simulink model "randomControllerSim2"  (R2015b)
settings: Solver=ode45  SolverMode=SingleTasking  StartTime=0.0  StopTime=2  RelTol=1e-3
values from neighbouring files (symbols this model uses):
  B_f = 7.4e-3    (= 0.0074)    [randomController.m]
  B_w = 17.03e-6    (= 1.703e-05)    [randomController.m]
  g = 9.82    [randomController.m]
  J_f = 5.6e-3    (= 0.0056)    [randomController.m]
  J_w = 0.601e-3    (= 0.000601)    [randomController.m]
  l_f = 0.08498    [randomController.m]
  l_w = 0.093    [randomController.m]
  m_f = 0.77-m_w    (= 0.548)    [randomController.m]
  m_w = 0.222    [randomController.m]
settings Model: Creator=USUARIO  LastModifiedBy=USUARIO
settings DataIOCC: SaveFormat=Array
settings OptimizationCC: BlockReduction=off  BooleanDataType=off
settings DebuggingCC: SaveWithParameterizedLinksMsg=none  UnderspecifiedInitializationDetection=Classic  MergeDetectMultiDrivingBlocksExec=none  SignalResolutionControl=TryResolveAllWithWarning
settings HardwareCC: ProdBitPerPointer=32  ProdLargestAtomicFloat=None  ProdIntDivRoundTo=Undefined  ProdEndianess=Unspecified  ProdWordSize=32  ProdHWDeviceType=32-bit Generic  TargetUnknown=on
settings GRTTargetCC: GeneratePreprocessorConditionals=Disable all
settings ConfigComp: CovModelRefEnable=Off  CovSFcnEnable=off

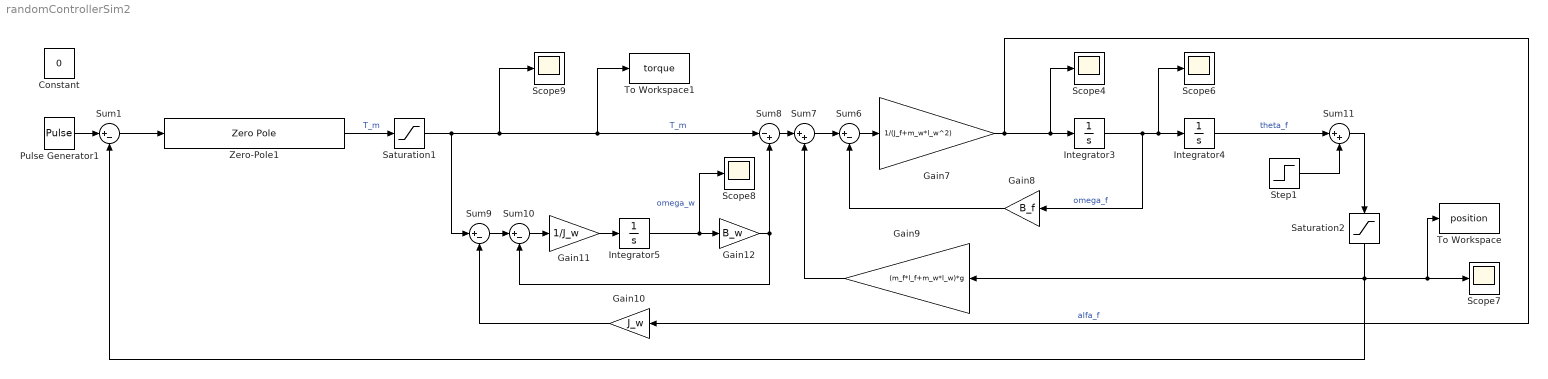
== system randomControllerSim2 ==
  Constant : Constant  Value=0
  Gain10 : Gain  Gain=J_w
  Gain11 : Gain  Gain=1/J_w
  Gain12 : Gain  Gain=B_w
  Gain7 : Gain  Gain=1/(J_f+m_w*l_w^2)
  Gain8 : Gain  Gain=B_f
  Gain9 : Gain  Gain=(m_f*l_f+m_w*l_w)*g
  Integrator3 : Integrator
  Integrator4 : Integrator
  Integrator5 : Integrator
  Pulse Generator1 : DiscretePulseGenerator  PulseType=Time based  Amplitude=-0.05  Period=10  PulseWidth=0.005
  Saturation1 : Saturate  UpperLimit=4*0.0335  LowerLimit=-4*0.0335
  Saturation2 : Saturate  UpperLimit=0.85  LowerLimit=-0.72
  Scope{4,6..9} (5 alike) : Scope
  Step1 : Step  Time=0.001  After=0  SampleTime=0
  Sum{1,6,9..10} (4 alike) : Sum  Inputs=|+-
  Sum11 : Sum  Inputs=|++
  Sum7 : Sum  Inputs=|++
  Sum8 : Sum  Inputs=|-+
  To Workspace : ToWorkspace  VariableName=position  SaveFormat=Timeseries  SampleTime=-1
  To Workspace1 : ToWorkspace  VariableName=torque  SaveFormat=Timeseries  SampleTime=-1
  Zero-Pole1 : ZeroPole  Zeros=[-9.483 -1.599]  Poles=[-200 -100 5.539]  Gain=[-0.62737*200*100*5.539/9.483/1.599]
  wires:
  Gain7/1 -> Gain10/1, Scope4/1, Integrator3/1  "alfa_f"
  Integrator3/1 -> Gain8/1, Scope6/1, Integrator4/1  "omega_f"
  Sum6/1 -> Gain7/1
  Sum7/1 -> Sum6/1
  Gain8/1 -> Sum6/2
  Gain9/1 -> Sum7/2
  Sum8/1 -> Sum7/1
  Sum10/1 -> Gain11/1
  Gain11/1 -> Integrator5/1
  Gain10/1 -> Sum9/2
  Sum9/1 -> Sum10/1
  Integrator5/1 -> Scope8/1, Gain12/1  "omega_w"
  Gain12/1 -> Sum10/2, Sum8/2
  Zero-Pole1/1 -> Saturation1/1  "T_m"
  Integrator4/1 -> Sum11/1  "theta_f"
  Step1/1 -> Sum11/2
  Sum1/1 -> Zero-Pole1/1
  Pulse Generator1/1 -> Sum1/1
  Sum11/1 -> Saturation2/1
  Saturation2/1 -> To Workspace/1, Scope7/1, Sum1/2, Gain9/1
  Saturation1/1 -> To Workspace1/1, Sum8/1, Scope9/1, Sum9/1  "T_m"
